simulink model "FSK_Implementation"  (R2021a)
settings: Solver=VariableStepAuto  StartTime=0.0  StopTime=10.0  RelTol=1e-3
libraries: commdigbbndfm2 x2, commchan3 x1, commsink2 x1, commsrccod2 x1, dspsigops x1, dspquant2 x1
settings Model: Creator=Bharat Gunhalkar  LastModifiedBy=Bharat Gunhalkar

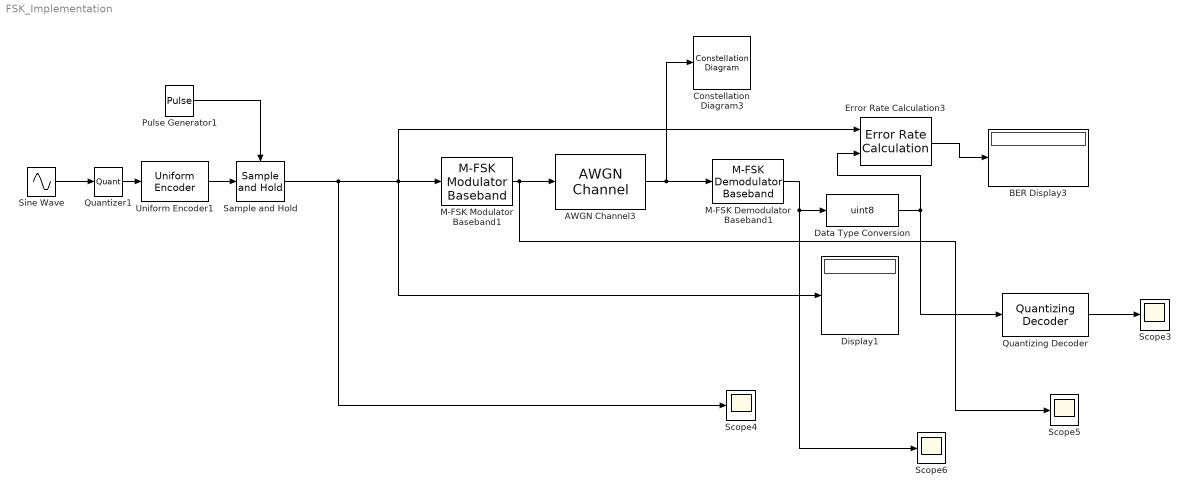
== system FSK_Implementation ==
  AWGN Channel3 : commchan3/AWGN Channel  InputProcessing=Columns as channels (frame based)  seed=67  noiseMode="Signal to noise ratio  (Eb/No)"  EbNodB=100  EsNodB=10  SNRdB=10  bitsPerSym=1  Ps=1  Tsym=1  variance=1
  BER Display3 : Display
  Constellation Diagram3 : ConstellationDiagram
  Data Type Conversion : DataTypeConversion  OutDataTypeStr=uint8
  Display1 : Display
  Error Rate Calculation3 : commsink2/Error Rate Calculation  N=0  st_delay=0  cp_mode=Entire frame  subframe=[]  PMode=Port  WsName=ErrorVec  RsMode2=off  stop=off  numErr=100  maxBits=1e6
  M-FSK Demodulator Baseband1 : commdigbbndfm2/M-FSK Demodulator Baseband  M=8  OutType=Integer  Dec=Gray  freqSep=6  numSamp=17  RateOptions=Enforce single-rate processing  outDataType=double
      settings: SourceProductBaseCode=CM
  M-FSK Modulator Baseband1 : commdigbbndfm2/M-FSK Modulator Baseband  M=8  InType=Integer  Enc=Gray  freqSep=6  phaseType=Continuous  numSamp=17  RateOptions=Enforce single-rate processing  outDataType=double
  Pulse Generator1 : DiscretePulseGenerator  SampleTime=0.001
  Quantizer1 : Quantizer  QuantizationInterval=.333
  Quantizing Decoder : commsrccod2/Quantizing Decoder  codebook=[-.825 -.5 0, .5 .825]  QuDType=double
      settings: SourceProductBaseCode=CM
  Sample and Hold : dspsigops/Sample and Hold  trig=Rising edge  initCond=0  latchinput=off
  Scope{3..6} (4 alike) : Scope
  Sine Wave : Sin  Amplitude=5  Frequency=2*pi  SampleTime=0.001
  Uniform Encoder1 : dspquant2/Uniform Encoder  peak=1  bits=3  otype=Unsigned integer
  wires:
  Quantizer1/1 -> Uniform Encoder1/1
  Sine Wave/1 -> Quantizer1/1
  Pulse Generator1/1 -> Sample and Hold/Trigger
  M-FSK Demodulator Baseband1/1 -> Scope6/1, Data Type Conversion/1
  Uniform Encoder1/1 -> Sample and Hold/1
  Error Rate Calculation3/1 -> BER Display3/1
  AWGN Channel3/1 -> M-FSK Demodulator Baseband1/1, Constellation Diagram3/1
  Quantizing Decoder/1 -> Scope3/1
  M-FSK Modulator Baseband1/1 -> Scope5/1, AWGN Channel3/1
  Sample and Hold/1 -> Scope4/1, Display1/1, Error Rate Calculation3/1, M-FSK Modulator Baseband1/1
  Data Type Conversion/1 -> Quantizing Decoder/1, Error Rate Calculation3/2
